simulink model "modify_scheme"  (R2023b)
settings: Solver=VariableStepAuto  StartTime=0.0  StopTime=10  RelTol=1e-3
StartFcn:
  | % Create a TCP/IP connection to the server
  | tcpObj = tcpclient('127.0.0.1', 8282);
StopFcn:
  | % Data to send
  | dataToSend = [-999, -999, -999, -999];
  | 
  | % Convert data to bytes. MATLAB uses doubles by default, so we explicitly ensure it's double.
  | % The 'typecast' function converts the double array into a uint8 byte array without changing the bit representation.
  | dataToSendBytes = typecast(double(dataToSend), 'double');
  | 
  | % Write data to the server
  | write(tcpObj, dataToSendBytes);
  | 
  | % Close the connection when done
  | clear tcpObj;
libraries: instrumentlib x2
settings Model: Creator=pc  LastModifiedBy=pc

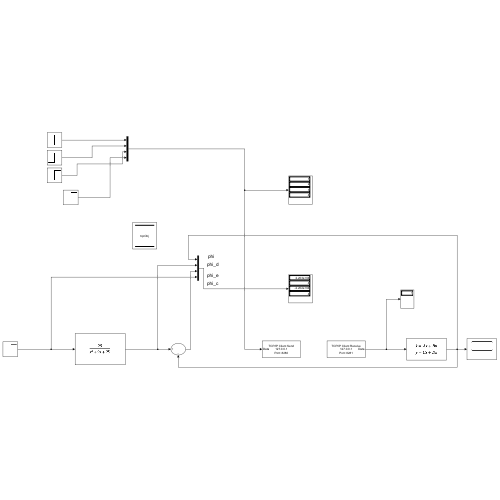
[thumbnail: Simulink's stored preview of the top-level diagram]
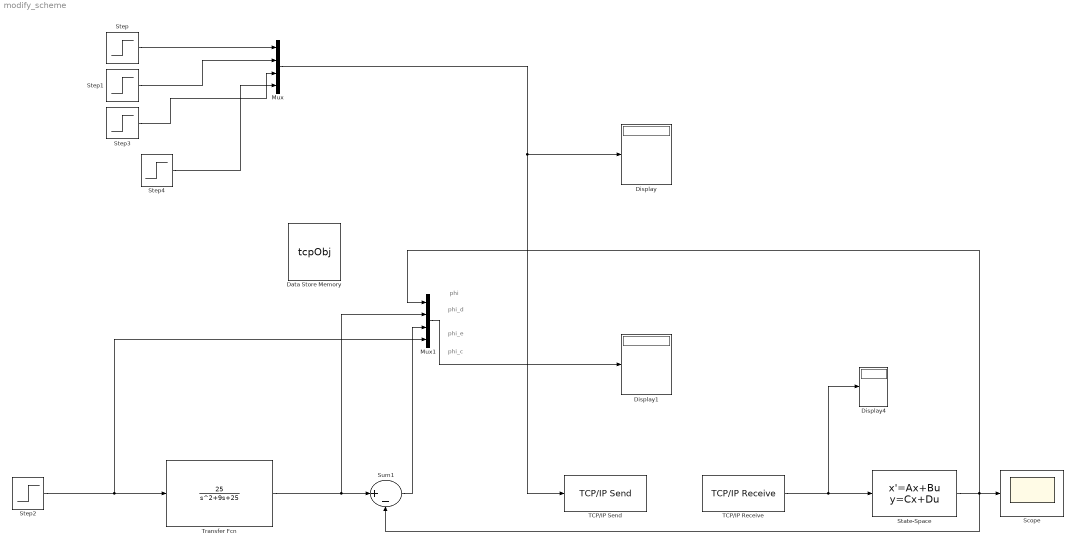
== system modify_scheme ==
  note: phi_c
  note: phi
  note: phi_d
  note: phi_e
  Data Store Memory : DataStoreMemory  DataStoreName=tcpObj  WriteAfterWriteMsg=warning  ShowAdditionalParam=off
  Display : Display
  Display1 : Display
  Display4 : Display
      settings: Decimation=3
  Mux : Mux
  Mux1 : Mux
  Scope : Scope
  State-Space : StateSpace  D=0  InitialCondition=0  ContinuousStateAttributes='Controlled_Object'
  Step : Step  Time=2  Before=1  SampleTime=0
  Step1 : Step  Time=2  Before=2  After=2  SampleTime=0
  Step2 : Step  Time=0  Before=4.0  After=4.0  SampleTime=0
  Step3 : Step  Time=2  Before=3  After=3  SampleTime=0
  Step4 : Step  Time=2  Before=4  After=4  SampleTime=0
  Sum1 : Sum  Inputs=|+-
  TCP/IP Receive : instrumentlib/TCP//IP Receive  Host=127.0.0.1  Port=8281  DataSize=[1]  DataType=double  ASCIIFormatting=%f  Terminator=LF  CustomTerminator=10  ByteOrder=big-endian  EnableBlockingMode=on  Timeout=10  SampleTime=0.01  SimulateUsing=Interpreted execution
  TCP/IP Send : instrumentlib/TCP//IP Send  Host=127.0.0.1  Port=8280  ByteOrder=big-endian  EnableBlockingMode=on  Timeout=10  TransferDelay=on  SimulateUsing=Interpreted execution
  Transfer Fcn : TransferFcn  StopFcn=|  Numerator=[25]  Denominator=[1 9 25]  ContinuousStateAttributes='Reference_Model'
      | % Create a TCP/IP connection to the server
      | tcpObj = tcpclient('127.0.0.1', 8280);
      | 
      | % Data to send
      | dataToSend = [-999, -999, -999, -999];
      | 
      | % Convert data to bytes if necessary. The conversion method depends on how the server expects to receive the data.
      | % Here, we'll assume the server expects four 32-bit integers in little-endian byte order.
      | dataToSendBytes = typecast(double(dataToSend), 'uint8');
      | 
      | % Write data to the server
      | write(tcpObj, dataToSendBytes);
      | 
      | % Close the connection when done
      | clear tcpObj;
  wires:
  Step4/1 -> Mux/4
  Step3/1 -> Mux/3
  Step1/1 -> Mux/2
  Step/1 -> Mux/1
  Mux/1 -> TCP/IP Send/1, Display/1
  Step2/1 -> Mux1/4, Transfer Fcn/1
  Transfer Fcn/1 -> Mux1/2, Sum1/1
  State-Space/1 -> Mux1/1, Sum1/2, Scope/1
  TCP/IP Receive/1 -> Display4/1, State-Space/1
  Sum1/1 -> Mux1/3
  Mux1/1 -> Display1/1
